simulink model "rigid_body_model"  (R2021a)
settings: Solver=ode4  StartTime=0  StopTime=10.0  FixedStep=T_sample_control  RelTol=1e-3  EnableMultiTasking=on
values from neighbouring files (symbols this model uses):
  x0 = 5000    [rigid_body_model.m]
libraries: vrlib x2, dspinverses x1
settings Model: DataDictionary=pid.sldd  EnableAccessToBaseWorkspace=off  ModifiedByFormat=The MathWorks Inc.  Creator=The MathWorks, Inc.  LastModifiedBy=The MathWorks Inc.
settings SolverCC: AlgebraicLoopSolver=TrustRegion
settings DataIOCC: SaveFormat=StructureWithTime  ReturnWorkspaceOutputs=off
settings OptimizationCC: BlockReduction=off  DefaultParameterBehavior=Inlined  InlineInvariantSignals=on  BufferReuse=off  PassReuseOutputArgsAs=Individual arguments  ExpressionDepthLimit=2147483647  ZeroExternalMemoryAtStartup=off  ZeroInternalMemoryAtStartup=off  EfficientFloat2IntCast=on  LifeSpan=1  EfficientTunableParamExpr=on
settings DebuggingCC: AlgebraicLoopMsg=none  FcnCallInpInsideContextMsg=warning  UnconnectedInputMsg=none  UnconnectedOutputMsg=none  UnconnectedLineMsg=none  UniqueDataStoreMsg=error  AssertControl=DisableAll  AllowSymbolicDim=off  StateNameClashWarn=warning  StrictBusMsg=ErrorOnBusTreatedAsVector  SFUnexpectedBacktrackingDiag=warning  SFNoUnconditionalDefaultTransitionDiag=warning  SFExecutionAtInitializationDiag=none  SFMachineParentedDataDiag=warning  ArithmeticOperatorsInVariantConditions=warning
settings HardwareCC: ProdBitPerPointer=32  ProdBitPerSizeT=32  ProdBitPerPtrDiffT=32  ProdLargestAtomicFloat=None  ProdIntDivRoundTo=Undefined  ProdEndianess=Unspecified  ProdWordSize=32  ProdHWDeviceType=32-bit Generic
settings ModelReferenceCC: PropagateSignalLabelsOutOfModel=off
settings SFSimCC: SimUseLocalCustomCode=off  CustomCodeUndefinedFunction=UseInterfaceOnly
settings RTWCC: SystemTargetFile=ert.tlc  TemplateMakefile=ert_default_tmf  GenerateReport=on  RTWUseLocalCustomCode=off  IncludeHyperlinkInReport=on  GenerateTraceInfo=on  GenerateTraceReport=on  GenerateTraceReportSl=on  GenerateTraceReportSf=on  GenerateTraceReportEml=on  GenerateCodeMetricsReport=on
settings CodeAppCC: IgnoreCustomStorageClasses=off  IgnoreTestpoints=on  CustomSymbolStrType=$N$R$M  StateflowObjectComments=on  InternalIdentifier=Classic
settings ERTTargetCC: MultiwordLength=2048  GenerateSampleERTMain=on  SupportNonFinite=off  ParenthesesLevel=Maximum  InlinedParameterPlacement=NonHierarchical  ERTCustomFileTemplate=example_file_process.tlc  ConvertIfToSwitch=off  SuppressUnreachableDefaultCases=off
settings ConfigComp: CovMetricSettings=dw  CovSaveCumulativeToWorkspaceVar=on  CovSaveSingleToWorkspaceVar=on  CovExternalEMLEnable=off  CovSFcnEnable=off

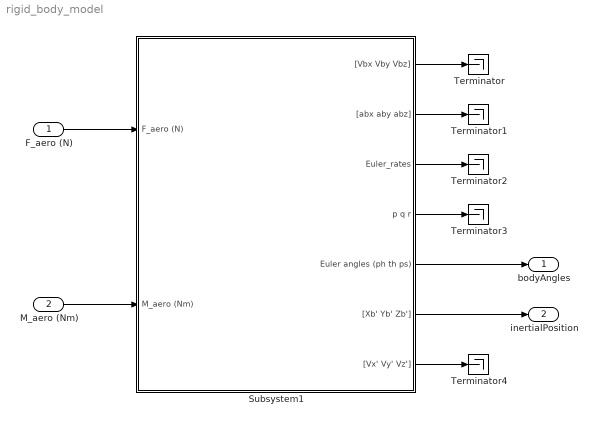
== system rigid_body_model ==
  F_aero (N) : Inport
  M_aero (Nm) : Inport  Port=2
  Subsystem1 : Subsystem
  Terminator{,1..4} (5 alike) : Terminator
  bodyAngles : Outport
  inertialPosition : Outport  Port=2
  wires:
  F_aero (N)/1 -> Subsystem1/1(F_aero (N))
  M_aero (Nm)/1 -> Subsystem1/2(M_aero (Nm))
  Subsystem1/5(Euler angles (ph th ps)) -> bodyAngles/1
  Subsystem1/6("[Xb' Yb' Zb']") -> inertialPosition/1
  Subsystem1/1("[Vbx Vby Vbz]") -> Terminator/1
  Subsystem1/2("[abx aby abz]") -> Terminator1/1
  Subsystem1/3(Euler_rates) -> Terminator2/1
  Subsystem1/4(p q r) -> Terminator3/1
  Subsystem1/7("[Vx' Vy' Vz']") -> Terminator4/1

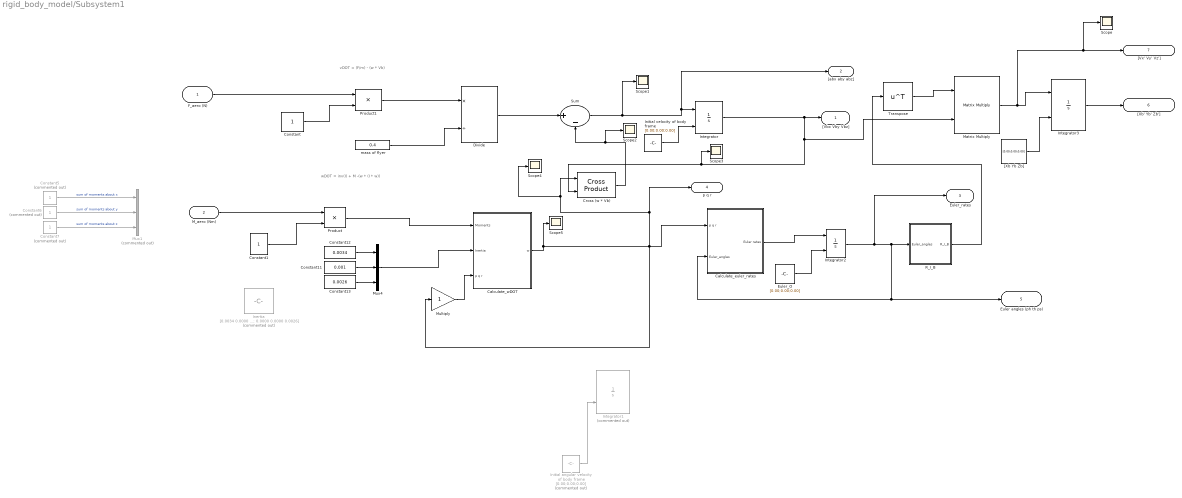
== system rigid_body_model/Subsystem1 ==
  note: wDOT = inv(I) + M -(w * (I * w))
  note: vDOT = (F/m) - (w * Vb)
  F_aero (N) : Inport
  M_aero (Nm) : Inport  Port=2
  Calculate_euler_rates : Subsystem
  Calculate_wDOT : Subsystem
  Constant : Constant
  Constant1 : Constant
  Constant11 : Constant  Value=0.001
  Constant12 : Constant  Value=0.0034
  Constant13 : Constant  Value=0.0026
  Constant5 : Constant  Commented=on
  Constant6 : Constant  Commented=on
  Constant7 : Constant  Commented=on
  Cross (w * Vb) : vrlib/Utilities/Cross Product
  Divide : Product  Inputs=*/
  Euler_O : Constant  Value=[0.00;0.00;0.00]
  Inertia : Constant  Commented=on  Value=[0.0034 0.0000 0.0000; 0.0000 0.0010 0.0000; 0.0000 0.0000 0.0026]
  Initial angular velocity of body frame : Constant  Commented=on  Value=[0.00;0.00;0.00]
  Initial velocity of body frame : Constant  Value=[0.00;0.00;0.00]
  Integrator : Integrator  InitialConditionSource=external  InitialCondition=x0
  Integrator1 : Integrator  Commented=on  InitialConditionSource=external
  Integrator2 : Integrator  InitialConditionSource=external
  Integrator3 : Integrator  InitialConditionSource=external
  Matrix Multiply : Product  Multiplication=Matrix(*)
  Multiply : Gain
  Mux1 : Mux  Commented=on  Inputs=3
  Mux4 : Mux  Inputs=3
  Product : Product
  Product1 : Product
  R_I_B : Subsystem
  Scope{,1..5} (6 alike) : Scope
  Sum : Sum  Inputs=|+-
  Transpose : Math  Operator=transpose  SaturateOnIntegerOverflow=on
  "[Xb Yb Zb]" : Constant  Value=[0.00;0.00;0.00]
  mass of flyer : Constant  Value=0.4
  "[Vbx Vby Vbz]" : Outport
  "[abx aby abz]" : Outport  Port=2
  Euler_rates : Outport  Port=3
  p q r : Outport  Port=4
  Euler angles (ph th ps) : Outport  Port=5
  "[Xb' Yb' Zb']" : Outport  Port=6
  "[Vx' Vy' Vz']" : Outport  Port=7
  wires:
  Euler_O/1 -> Integrator2/2
  Initial velocity of body frame/1 -> Integrator/2
  Product/1 -> Calculate_wDOT/1(Moments)
  Calculate_euler_rates/1(Euler rates) -> Integrator2/1
  Initial angular velocity of body frame/1 -> Integrator1/2
  R_I_B/1(R_I_B) -> Transpose/1
  F_aero (N)/1 -> Product1/1
  Constant12/1 -> Mux4/1
  Product1/1 -> Divide/1
  Constant13/1 -> Mux4/3
  Calculate_wDOT/1(w) -> Multiply/1, Scope4/1, Cross (w * Vb)/1, p q r/1, Calculate_euler_rates/1(p q r), Scope5/1
  Transpose/1 -> Matrix Multiply/1
  Constant7/1 -> Mux1/3  "sum of moments about z"
  Divide/1 -> Sum/1
  "[Xb Yb Zb]"/1 -> Integrator3/2
  Constant/1 -> Product1/2
  mass of flyer/1 -> Divide/2
  Multiply/1 -> Calculate_wDOT/3(p q r)
  Mux4/1 -> Calculate_wDOT/2(Inertia)
  Matrix Multiply/1 -> Scope/1, "[Vx' Vy' Vz']"/1, Integrator3/1
  Constant1/1 -> Product/2
  Integrator/1 -> "[Vbx Vby Vbz]"/1, Scope3/1, Cross (w * Vb)/2, Matrix Multiply/2
  Integrator3/1 -> "[Xb' Yb' Zb']"/1
  Constant11/1 -> Mux4/2
  M_aero (Nm)/1 -> Product/1
  Cross (w * Vb)/1 -> Scope2/1, Sum/2
  Integrator2/1 -> Euler_rates/1, Calculate_euler_rates/2(Euler_angles), Euler angles (ph th ps)/1, R_I_B/1(Euler_angles)
  Constant6/1 -> Mux1/2  "sum of moments about y"
  Sum/1 -> Scope1/1, "[abx aby abz]"/1, Integrator/1
  Constant5/1 -> Mux1/1  "sum of moments about x"

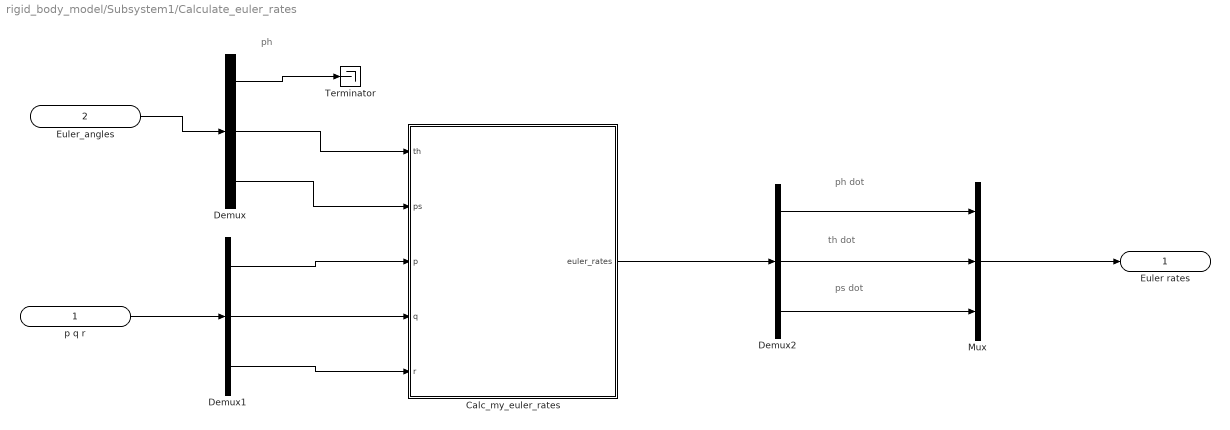
== system rigid_body_model/Subsystem1/Calculate_euler_rates ==
  note: ps dot
  note: th dot
  note: ph dot
  note: ph
  p q r : Inport
  Euler_angles : Inport  Port=2
  Calc_my_euler_rates : MATLAB Function  TreatAsAtomicUnit=on
  Demux : Demux  Outputs=[-1;1;1]
  Demux1 : Demux  Outputs=[1;1;1]
  Demux2 : Demux  Outputs=3
  Mux : Mux  Inputs=3
  Terminator : Terminator
  Euler rates : Outport
  wires:
  Demux/1 -> Terminator/1
  Euler_angles/1 -> Demux/1
  Demux/2 -> Calc_my_euler_rates/1(th)
  Demux/3 -> Calc_my_euler_rates/2(ps)
  p q r/1 -> Demux1/1
  Demux1/2 -> Calc_my_euler_rates/4(q)
  Demux1/1 -> Calc_my_euler_rates/3(p)
  Demux1/3 -> Calc_my_euler_rates/5(r)
  Calc_my_euler_rates/1(euler_rates) -> Demux2/1
  Demux2/2 -> Mux/2
  Demux2/1 -> Mux/1
  Demux2/3 -> Mux/3
  Mux/1 -> Euler rates/1

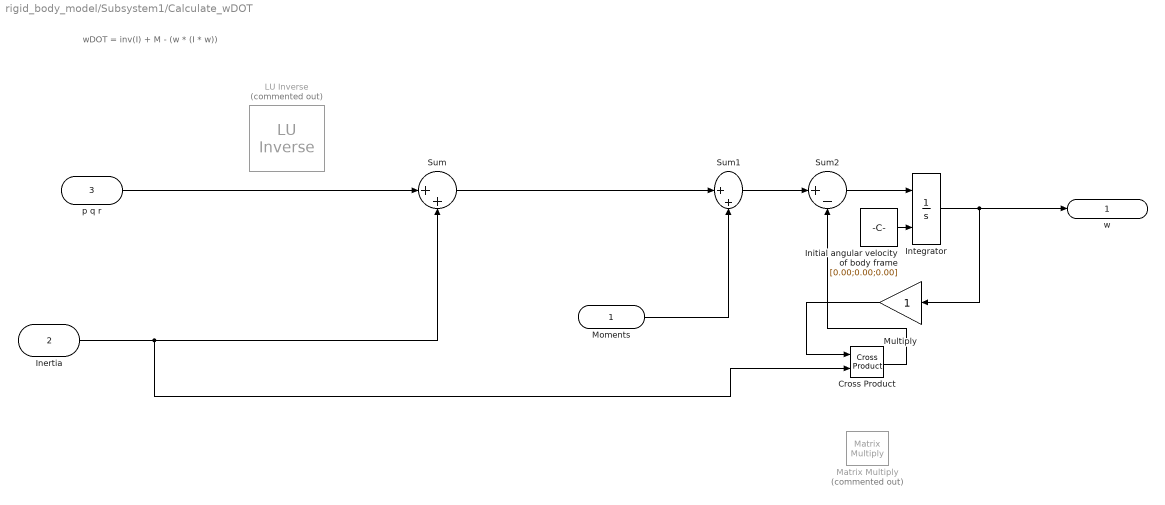
== system rigid_body_model/Subsystem1/Calculate_wDOT ==
  note: wDOT = inv(I) + M - (w * (I * w))
  Moments : Inport
  Inertia : Inport  Port=2
  p q r : Inport  Port=3
  " LU Inverse" : dspinverses/ LU Inverse  Commented=on
  Cross Product : vrlib/Utilities/Cross Product
  Initial angular velocity of body frame : Constant  Value=[0.00;0.00;0.00]
  Integrator : Integrator  InitialConditionSource=external
  Matrix Multiply : Product  Commented=on  Multiplication=Matrix(*)
  Multiply : Gain
  Sum : Sum  Inputs=|++
  Sum1 : Sum  Inputs=|++
  Sum2 : Sum  Inputs=|+-
  w : Outport
  wires:
  Sum/1 -> Sum1/1
  Sum1/1 -> Sum2/1
  Sum2/1 -> Integrator/1
  Cross Product/1 -> Sum2/2
  Integrator/1 -> Multiply/1, w/1
  Moments/1 -> Sum1/2
  p q r/1 -> Sum/1
  Inertia/1 -> Cross Product/2, Sum/2
  Multiply/1 -> Cross Product/1
  Initial angular velocity of body frame/1 -> Integrator/2

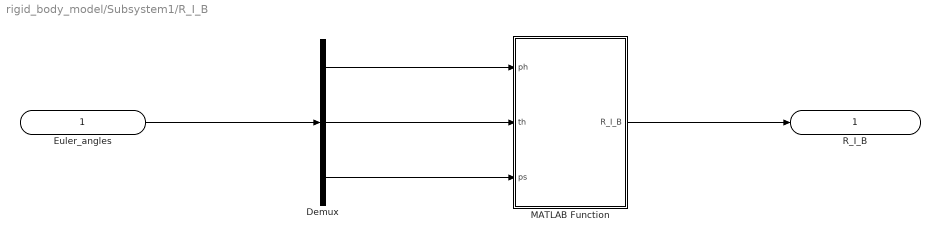
== system rigid_body_model/Subsystem1/R_I_B ==
  Euler_angles : Inport
  Demux : Demux  Outputs=[1;1;1]
  MATLAB Function : MATLAB Function  TreatAsAtomicUnit=on
  R_I_B : Outport
  wires:
  Euler_angles/1 -> Demux/1
  Demux/2 -> MATLAB Function/2(th)
  Demux/3 -> MATLAB Function/3(ps)
  Demux/1 -> MATLAB Function/1(ph)
  MATLAB Function/1(R_I_B) -> R_I_B/1

== matlab function rigid_body_model/Subsystem1/Calculate_euler_rates/Calc_my_euler_rates ==
  data: th input; euler_rates output; ps input; p input; q input; r input
function euler_rates = my_euler_rates(th,ps,p,q,r)
euler_rates = [(r .* cos(ps) + q .* sin(ps)) ./ cos(th);
                q .* cos(ps) - r .* sin(ps);
                (p .* cos(th) + r.* cos(ps) .* sin(th) + q .* sin(ps) .* sin(th)) ./ cos(th)];
end

== matlab function rigid_body_model/Subsystem1/R_I_B/MATLAB Function ==
  data: ph input; R_I_B output; th input; ps input
function R_I_B = calc_R_I_B(ph, th, ps)

R_I_B = [cos(th)*cos(ps)              cos(th)*sin(ps)              -sin(th);
               sin(ph)*sin(th)*cos(ps)-cos(ph)*sin(ps)  sin(ph)*sin(th)*sin(ps)+cos(ph)*cos(ps)  sin(ph)*cos(th);
               cos(ph)*sin(th)*cos(ps)+sin(ph)*sin(ps)  cos(ph)*sin(th)*sin(ps)-sin(ph)*cos(ps)  cos(ph)*cos(th)];
end
